simulink model "t9_masa_amortiguador_resorte"  (R2024a)
settings: Solver=ode23t  StartTime=0.0  StopTime=5  FixedStep=0.001  RelTol=1e-3  AbsTol=1e-3
libraries: fl_lib x8, nesl_utility x3
settings Model: Creator=jibmo  LastModifiedBy=scpmoxxa
settings SolverCC: AutoScaleAbsTol=off  AlgebraicLoopSolver=TrustRegion  MaxZcPerStep=1
settings OptimizationCC: ReuseModelBlockBuffer=off
settings DebuggingCC: UnconnectedInputMsg=warning  UnconnectedOutputMsg=warning  UnconnectedLineMsg=warning  SymbolicDimsDataTypeCodeGenerationDiagnostic=none
settings ModelReferenceCC: EnableRefExpFcnMdlSchedulingChecks=on
settings SFSimCC: CustomCodeUndefinedFunction=UseInterfaceOnly
settings RTWCC: GPUComputeCapability=3.5  DLArmComputeVersion=19.05
settings SimscapeCC: SimscapeLogType=all  SimscapeLogSimulationStatistics=on  SimscapeLogDataHistory=10000

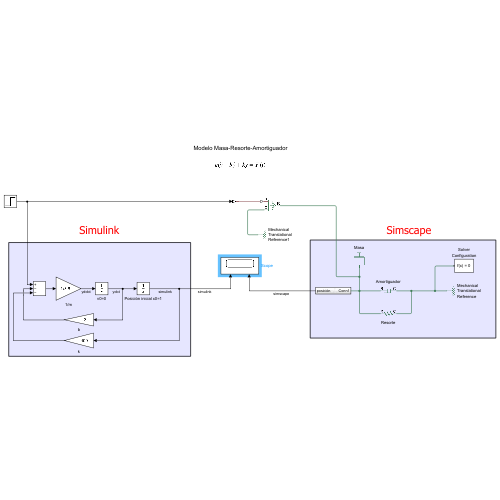
[thumbnail: Simulink's stored preview of the top-level diagram]
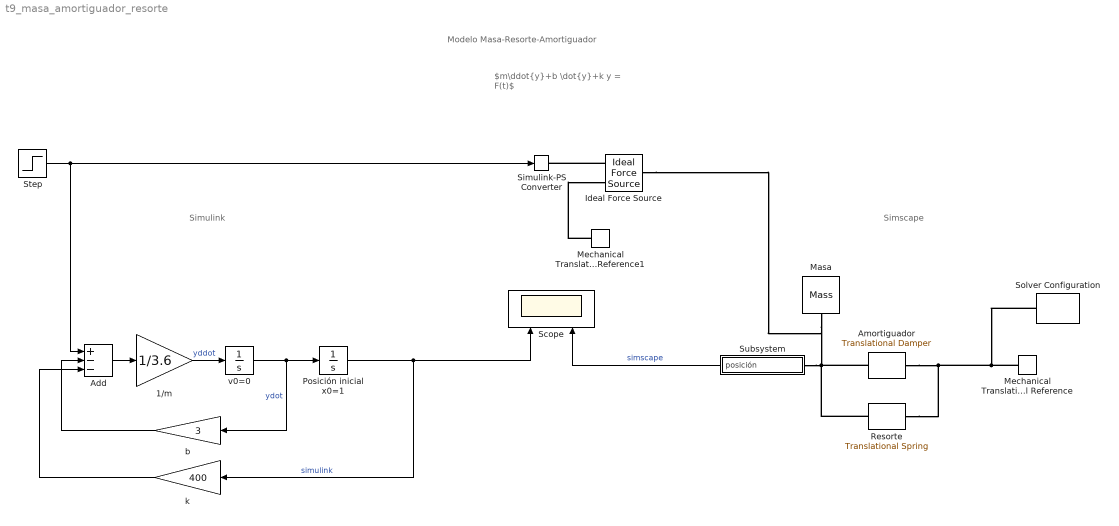
== system t9_masa_amortiguador_resorte ==
  note: Simulink
  note: Modelo Masa-Resorte-Amortiguador
  note: $m\ddot{y}+b \dot{y}+k y = F(t)$
  note: Simscape
  1/m : Gain  SCDEnableBlockLinearizationSpecification=on  Gain=1/3.6
  Add : Sum  Inputs=+--
  Amortiguador : fl_lib/Mechanical/Translational Elements/Translational Damper  D=3 N*s/m  v_specify=off  v_priority=None  v=0 m/s  v_nominal_specify=off  v_nominal_value=1  v_nominal_unit=m/s  f_specify=off  f_priority=None  f=0 N  f_nominal_specify=off  f_nominal_value=1  f_nominal_unit=N
  Ideal Force Source : fl_lib/Mechanical/Mechanical Sources/Ideal Force Source
  Masa : fl_lib/Mechanical/Translational Elements/Mass  mass=3.6 kg  num_ports=foundation.enum.numPorts2.one  v_specify=off  v_priority=High  v=15 m/s  v_nominal_specify=off  v_nominal_value=1  v_nominal_unit=m/s  f_specify=off  f_priority=None  f=1 N  f_nominal_specify=off  f_nominal_value=1  f_nominal_unit=N
  Mechanical Translational Reference : fl_lib/Mechanical/Translational Elements/Mechanical Translational Reference
  Mechanical Translational Reference1 : fl_lib/Mechanical/Translational Elements/Mechanical Translational Reference
  Posición inicial x0=1 : Integrator  InitialCondition=1
  Resorte : fl_lib/Mechanical/Translational Elements/Translational Spring  spr_rate=400 N/m  v_specify=off  v_priority=None  v=0 m/s  v_nominal_specify=off  v_nominal_value=1  v_nominal_unit=m/s  f_specify=off  f_priority=None  f=0 N  f_nominal_specify=off  f_nominal_value=1  f_nominal_unit=N  x_specify=on  x_priority=High  x=1 m  x_nominal_specify=on  x_nominal_value=1  x_nominal_unit=m
  Scope : Scope  NumInputPorts=2
  Simulink-PS Converter : nesl_utility/Simulink-PS Converter  PhysicalDomain=network_engine_domain  SubClassName=ps_input  LeftPortType=input  RightPortType=output  PseudoPeriodic=off  Frequencies=[]  NoiseDistribution=none  NoiseParameters=[]  Unit=1  AffineConversion=off  FilteringAndDerivatives=provide  SimscapeFilterOrder=1  InputFilterTimeConstant=0.001  UdotUserProvided=0
  Solver Configuration : nesl_utility/Solver Configuration  PhysicalDomain=network_engine_domain  SubClassName=solver  LeftPortType=input  RightPortType=generic  Tones=[]  Harmonics=[]  SimulateNoise=off  Profile=off  UseLocalSampling=off  EnableSwitchedLinearOptims=on  FrequencyDomain=off  UseCCode=off  RelTol=0.001  AbsTol=1e-06  MinStep=1e-09  ToWorkspace=off  RevertToSquareIcSolve=off  NumHomotopyIterations=100  PhasorMode=off  PhasorModeNumHarmonics=1  ConsistencySolver=NEWTON_XTOL_AFTER_FTOL  IndexReductionMethod=DerivativeReplacement  DoDC=off  ResidualTolerance=1e-09  ConsistencyTolSource=LOCAL  ConsistencyAbsTol=0.001  ConsistencyRelTol=0.001  ConsistencyTolFactor=0.001  UseLocalSolver=off  LocalSolverChoice=NE_TRAPEZOIDAL_ADVANCER  ResolveIndetEquations=on  FunctionEvalNumThread=1  LocalSolverSampleTime=0.001  DoFixedCost=off  MaxNonlinIter=3  MaxModeIter=2  ComputeImpulses=off  ImpulseIterations=2  LinearAlgebra=auto  LinearAlgebraNumThread=0  EquationFormulation=NE_TIME_EF  DelaysMemoryBudget=1024  AutomaticFiltering=on  FilteringTimeConstant=0.001  PartitionStorageMethod=AS_NEEDED  PartitionMemoryBudget=1024  PartitionMethod=ROBUST  MultibodyUseLocalSolver=off  MultibodyLocalSolverChoice=ODE1  MultibodyLocalSolverSampleTime=0.001
  Step : Step  Time=.1  After=100  SampleTime=0
  Subsystem : Subsystem
  b : Gain  SCDEnableBlockLinearizationSpecification=on  Gain=3
  k : Gain  SCDEnableBlockLinearizationSpecification=on  Gain=400
  v0=0 : Integrator
  wires:
  Posición inicial x0=1/1 -> Scope/1, k/1  "simulink"
  b/1 -> Add/2
  v0=0/1 -> b/1, Posición inicial x0=1/1  "ydot"
  Add/1 -> 1/m/1
  1/m/1 -> v0=0/1  "yddot"
  Subsystem/1(posición) -> Scope/2  "simscape"
  Step/1 -> Add/1, Simulink-PS Converter/1
  k/1 -> Add/3
  connections:
  Solver Configuration/RConn1 -- Mechanical Translational Reference/LConn1 -- Resorte/RConn1 -- Amortiguador/RConn1
  Resorte/LConn1 -- Ideal Force Source/LConn1 -- Masa/LConn1 -- Subsystem/LConn1 -- Amortiguador/LConn1
  Ideal Force Source/RConn1 -- Simulink-PS Converter/RConn1
  Mechanical Translational Reference1/LConn1 -- Ideal Force Source/RConn2

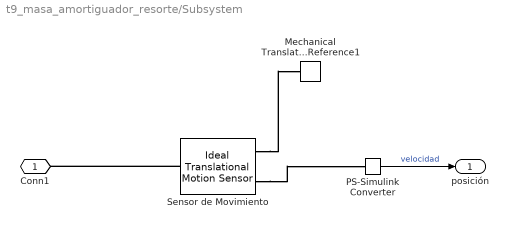
== system t9_masa_amortiguador_resorte/Subsystem ==
  Mechanical Translational Reference1 : fl_lib/Mechanical/Translational Elements/Mechanical Translational Reference
  PS-Simulink Converter : nesl_utility/PS-Simulink Converter  PhysicalDomain=network_engine_domain  SubClassName=ps_output  LeftPortType=input  RightPortType=output  PseudoPeriodic=off  Frequencies=[]  VectorFormat=inherit  Unit=inherit  AffineConversion=off
  Sensor de Movimiento : fl_lib/Mechanical/Mechanical Sensors/Ideal Translational Motion Sensor  reference=foundation.enum.MeasurementReference.difference  acceleration_port=false  velocity_port=false  position_port=true  offset=1 m
      settings: InternalSimscapePortConfiguration="{\"Bottom\":[],\"Left\":[{\"id\":\"R\",\"label\":\"R\",\"type\":\"foundation.mechanical.translational.translational\"}],\"Right\":[{\"id\":\"C\",\"label\":\"C\",\"type\":\"foundation.mechanical.translational.translational\"},{\"id\":\"P\",\"label\":\"P\",\"type\":\"output\"}],\"Top\":[]}"
  Conn1 : PMIOPort  Side=Left
  posición : Outport
  wires:
  PS-Simulink Converter/1 -> posición/1  "velocidad"
  connections:
  Sensor de Movimiento/RConn1 -- Mechanical Translational Reference1/LConn1
  Sensor de Movimiento/RConn2 -- PS-Simulink Converter/LConn1
  Sensor de Movimiento/LConn1 -- Conn1/RConn1
